simulink model "SWC_HALOUT_type"  (R2021b)
settings: Solver=FixedStepDiscrete  StartTime=0.0  StopTime=10.0  FixedStep=0.001  RelTol=1e-3
values from neighbouring files (symbols this model uses):
  DIDLen_APPPedalZP = uint16(3)    [vcu_local_hdr.m]
  DIDLen_APSFunConfig = uint16(16)    [vcu_local_hdr.m]
  DIDLen_AutoLock = uint16(1)    [vcu_local_hdr.m]
  DIDLen_AutoWipHSpdEN = uint16(1)    [vcu_local_hdr.m]
  DIDLen_DKCKey = uint16(8)    [vcu_local_hdr.m]
  DIDLen_DRLDis = uint16(1)    [vcu_local_hdr.m]
  DIDLen_DynoMode = uint16(1)    [vcu_local_hdr.m]
  DIDLen_FMHTimer = uint16(1)    [vcu_local_hdr.m]
  DIDLen_LFLowPresThre = uint16(1)    [vcu_local_hdr.m]
  DIDLen_LFSensorID = uint16(4)    [vcu_local_hdr.m]
  DIDLen_LRLowPresThre = uint16(1)    [vcu_local_hdr.m]
  DIDLen_LRSensorID = uint16(4)    [vcu_local_hdr.m]
  DIDLen_NVMPedalZP = uint16(3)    [vcu_local_hdr.m]
  DIDLen_RFLowPresThre = uint16(1)    [vcu_local_hdr.m]
  DIDLen_RFSensorID = uint16(4)    [vcu_local_hdr.m]
  DIDLen_RRLowPresThre = uint16(1)    [vcu_local_hdr.m]
  DIDLen_RRSensorID = uint16(4)    [vcu_local_hdr.m]
  DIDLen_SensorMode = uint16(1)    [vcu_local_hdr.m]
  DIDLen_TireSize = uint16(16)    [vcu_local_hdr.m]
  DIDLen_TPMSLearnSta = uint16(1)    [vcu_local_hdr.m]
  DIDLen_TurnLampFLThreCurr = uint16(1)    [vcu_local_hdr.m]
  DIDLen_TurnLampFRThreCurr = uint16(1)    [vcu_local_hdr.m]
  DIDLen_TurnLampRLThreCurr = uint16(1)    [vcu_local_hdr.m]
  DIDLen_TurnLampRRThreCurr = uint16(1)    [vcu_local_hdr.m]
  DIDLen_USSConfig = uint16(16)    [vcu_local_hdr.m]
  DIDLen_WhlPres = uint16(4)    [vcu_local_hdr.m]
  DIDLen_WhlSensorBattSta = uint16(1)    [vcu_local_hdr.m]
  DIDLen_WhlTmp = uint16(4)    [vcu_local_hdr.m]
  DIDLen_WipRLSCmdCutFilter = uint16(1)    [vcu_local_hdr.m]
  DIDLen_WipRLSCmdHoldFilter = uint16(1)    [vcu_local_hdr.m]
  DIDLen_XWDMode = uint16(1)    [vcu_local_hdr.m]
  DIDNum_APPPedalZP = uint16(0x0206)    [vcu_local_hdr.m]
  DIDNum_APSFunConfig = uint16(0x0903)    [vcu_local_hdr.m]
  DIDNum_AutoLock = uint16(0x0306)    [vcu_local_hdr.m]
  DIDNum_AutoWipHSpdEN = uint16(0x0308)    [vcu_local_hdr.m]
  DIDNum_DKCKey = uint16(0x0202)    [vcu_local_hdr.m]
  DIDNum_DRLDis = uint16(0x0307)    [vcu_local_hdr.m]
  DIDNum_DynoMode = uint16(0x0203)    [vcu_local_hdr.m]
  DIDNum_FMHTimer = uint16(0x0305)    [vcu_local_hdr.m]
  DIDNum_LFLowPresThre = uint16(0x0B08)    [vcu_local_hdr.m]
  DIDNum_LFSensorID = uint16(0x0B01)    [vcu_local_hdr.m]
  DIDNum_LRLowPresThre = uint16(0x0B0A)    [vcu_local_hdr.m]
  DIDNum_LRSensorID = uint16(0x0B03)    [vcu_local_hdr.m]
  DIDNum_NVMPedalZP = uint16(0x0207)    [vcu_local_hdr.m]
  DIDNum_RFLowPresThre = uint16(0x0B09)    [vcu_local_hdr.m]
  DIDNum_RFSensorID = uint16(0x0B02)    [vcu_local_hdr.m]
  DIDNum_RRLowPresThre = uint16(0x0B0B)    [vcu_local_hdr.m]
  DIDNum_RRSensorID = uint16(0x0B04)    [vcu_local_hdr.m]
  DIDNum_SensorMode = uint16(0x0B0C)    [vcu_local_hdr.m]
  DIDNum_TireSize = uint16(0x0902)    [vcu_local_hdr.m]
  DIDNum_TPMSLearnSta = uint16(0x0B0D)    [vcu_local_hdr.m]
  DIDNum_TurnLampFLThreCurr = uint16(0x0303)    [vcu_local_hdr.m]
  DIDNum_TurnLampFRThreCurr = uint16(0x0301)    [vcu_local_hdr.m]
  DIDNum_TurnLampRLThreCurr = uint16(0x0304)    [vcu_local_hdr.m]
  DIDNum_TurnLampRRThreCurr = uint16(0x0302)    [vcu_local_hdr.m]
  DIDNum_USSConfig = uint16(0x0901)    [vcu_local_hdr.m]
  DIDNum_WhlPres = uint16(0x0B05)    [vcu_local_hdr.m]
  DIDNum_WhlSensorBattSta = uint16(0x0B07)    [vcu_local_hdr.m]
  DIDNum_WhlTmp = uint16(0x0B06)    [vcu_local_hdr.m]
  DIDNum_WipRLSCmdCutFilter = uint16(0x030A)    [vcu_local_hdr.m]
  DIDNum_WipRLSCmdHoldFilter = uint16(0x0309)    [vcu_local_hdr.m]
  DIDNum_XWDMode = uint16(0x0201)    [vcu_local_hdr.m]
  ENUM_TPMSLearnStatus_LEARNED = uint8(  1  )    [vcu_local_hdr.m]
  ENUM_TPMSLearnStatus_LEARNFAIL = uint8(  2  )    [vcu_local_hdr.m]
  ENUM_TPMSLearnStatus_NOTLEARN = uint8(  0  )    [vcu_local_hdr.m]
  FALSE = boolean( 0 )    [vcu_local_hdr.m]    (also in vcu_local_hdrTA2.m)
  TRUE = boolean( 1 )    [vcu_local_hdr.m]    (also in vcu_local_hdrTA2.m)
  ZERO_INT = uint8(0)    [vcu_local_hdr.m]    (also in vcu_local_hdrTA2.m)
undefined symbols (not defined in the file or in its folder): f32_ApsOutVehSpdSig, R_DIDWriteCDD_CSOP_DIDSet_APPPedalZP, R_DIDWriteCDD_CSOP_DIDSet_APSFunConfig, R_DIDWriteCDD_CSOP_DIDSet_AutoLock, R_DIDWriteCDD_CSOP_DIDSet_AutoWipHSpdEN, R_DIDWriteCDD_CSOP_DIDSet_DKCKey, R_DIDWriteCDD_CSOP_DIDSet_DRLDis, R_DIDWriteCDD_CSOP_DIDSet_DynoMode, R_DIDWriteCDD_CSOP_DIDSet_FMHTimer, R_DIDWriteCDD_CSOP_DIDSet_LFLowPresThre, R_DIDWriteCDD_CSOP_DIDSet_LFSensorID, R_DIDWriteCDD_CSOP_DIDSet_LRLowPresThre, R_DIDWriteCDD_CSOP_DIDSet_LRSensorID, R_DIDWriteCDD_CSOP_DIDSet_NVMPedalZP, R_DIDWriteCDD_CSOP_DIDSet_RFLowPresThre, R_DIDWriteCDD_CSOP_DIDSet_RFSensorID, R_DIDWriteCDD_CSOP_DIDSet_RRLowPresThre, R_DIDWriteCDD_CSOP_DIDSet_RRSensorID, R_DIDWriteCDD_CSOP_DIDSet_SensorMode, R_DIDWriteCDD_CSOP_DIDSet_TireSize, R_DIDWriteCDD_CSOP_DIDSet_TPMSLearnSta, R_DIDWriteCDD_CSOP_DIDSet_TurnLampFLThreCurr, R_DIDWriteCDD_CSOP_DIDSet_TurnLampFRThreCurr, R_DIDWriteCDD_CSOP_DIDSet_TurnLampRLThreCurr, R_DIDWriteCDD_CSOP_DIDSet_TurnLampRRThreCurr, R_DIDWriteCDD_CSOP_DIDSet_USSConfig, R_DIDWriteCDD_CSOP_DIDSet_WhlPres, R_DIDWriteCDD_CSOP_DIDSet_WhlSensorBattSta, R_DIDWriteCDD_CSOP_DIDSet_WhlTmp, R_DIDWriteCDD_CSOP_DIDSet_WipRLSCmdCutFilter, R_DIDWriteCDD_CSOP_DIDSet_WipRLSCmdHoldFilter, R_DIDWriteCDD_CSOP_DIDSet_XWDMode, R_FDCCDD_Inner_CSOP_FDC_AppCallSleep, R_HALINCDD_CSOP_PAS_Handler, R_HALINCDD_CSOP_UDS_Main, R_HALOUT_APS_CSOP_ApsOutput, R_HALOUTCDD_CSOP_AppNmStateReq, R_HALOUTCDD_CSOP_ResetPedalZeroPosDone, R_HALOUTCDD_CSOP_SetAcoreRebootCmdACK, R_HALOUTCDD_CSOP_SetHazardIND, R_HALOUTCDD_CSOP_SetSysPwrStat, R_HALOUTCDD_CSOP_SleepRequest, R_HALOUTCDD_CSOP_TPMSSensorIDRegSetResults, R_IOExpOUT_CDD_CSOP_IOExpSetVal, R_J1939_CAN1_FD1_CE100_0_CSOP_Write_CAN1_FD1_CE100_0, R_J1939_CAN1_FD1_CE100_1_CSOP_Write_CAN1_FD1_CE100_1, R_NVMWriteCDD_Inner_NVM_WriteOperation, R_UDSCDD_CSOP_DdmRestartOperationCycle, R_WDGCDD_CSOP_Call_WDG_AppEnd, u16_DIDLen_APPPedalZP, u16_DIDLen_APSFunConfig, u16_DIDLen_AutoLock, u16_DIDLen_AutoWipHSpdEN, u16_DIDLen_DKCKey, u16_DIDLen_DRLDis, u16_DIDLen_DynoMode, u16_DIDLen_FMHTimer, u16_DIDLen_LFLowPresThre, u16_DIDLen_LFSensorID, u16_DIDLen_LRLowPresThre ... (+95)
libraries: FVT_lib x142, simulink x107, hdlsllib x6, hcu_lib x5, halout x1
(part 6 of 8)

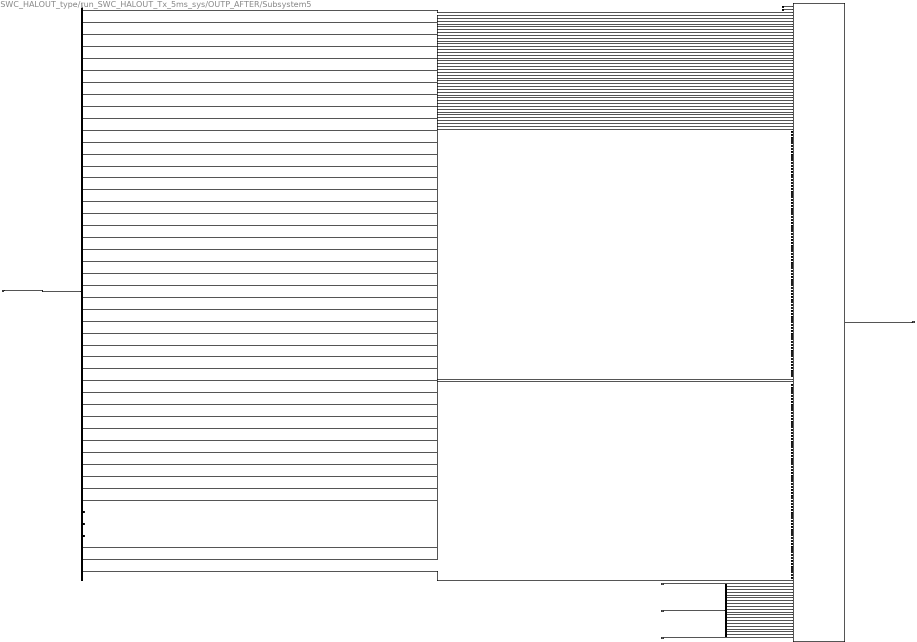
== system SWC_HALOUT_type/run_SWC_HALOUT_Tx_5ms_sys/OUTP_AFTER/Subsystem5 ==
  BOUTP_outputs : Inport
  BHAL_SYSTPMS_outputs : Inport  Port=2
  BHAL_SYS_outputs : Inport  Port=3
  BHAL_DIDGetData_raw : Inport  Port=4
  Bus Selector : BusSelector  OutputSignals=VOUTP_WriteChkLFID_raw,VOUTP_WriteChkRFID_raw,VOUTP_WriteChkLRID_raw,VOUTP_WriteChkRRID_raw,VOUTP_WriteChkfinLFID_raw,VOUTP_WriteChkfinRFID_raw,VOUTP_WriteChkfinLRID_raw,VOUTP_WriteChkfinRRID_raw,VOUTP_LFSensorFail_flg,VOUTP_RFSensorFail_flg,VOUTP_LRSensorFail_flg,VOUTP_RRSensorFail_flg,VOUTP_LFWheelPSW_raw8,VOUTP_RFWheelPSW_raw8,VOUTP_LRWheelPSW_raw8,VOUTP_RRWheelPSW_raw8,VOUTP_LFPindi_enum,VOUTP_RFPind_enum,VOUTP_LRPindi_enum,VOUTP_RRPindi_enum,VOUTP_LFP20_raw8,VOUTP_RFP20_raw8,VOUTP_LRP20_raw8,VOUTP_RRP20_raw8,VOUTP_LFWheelPress_raw8,VOUTP_RFWheelPress_raw8,VOUTP_LRWheelPress_raw8,VOUTP_RRWheelPress_raw8,VOUTP_LFWheelTemp_C,VOUTP_RFWheelTemp_C,VOUTP_LRWheelTemp_C,VOUTP_RRWheelTemp_C,VOUTP_Flashchkdatavalid_enum,VOUTP_Flashdatavalid_enum,VOUTP_unlearnSfali_flg,VOUTP_unlearnSfailvalid_enum,VOUTP_Prepresstempvalid_enum,VOUTP_FlashS1ID_raw,VOUTP_FlashS2ID_raw,VOUTP_FlashS3ID_raw,VOUTP_FlashS4ID_raw,VOUTP_FlashIDvalid_enum,VOUTP_EAPS1MIN_pct,VOUTP_EAPS2MIN_pct,VOUTP_SaveRegenMode_enum,VOUTP_ModelVersion_raw,VOUTP_ModelVersionChksum_raw,VOUTP_JudgeKeepUnlockZone_flg
  Bus Selector1 : BusSelector  OutputSignals=VHAL_RandomnumberY_raw1,VHAL_RandomnumberY_raw2,VHAL_RandomnumberY_raw3,VHAL_RandomnumberY_raw4,VHAL_RandomnumberY_raw5,VHAL_RandomnumberY_raw6,VHAL_RandomnumberY_raw7,VHAL_RandomnumberY_raw8,VHAL_funAuto_flg,VHAL_DiagDRLOFF_flg,VHAL_DiagFMHT_s,VHAL_DiagFLTC_mA,VHAL_DiagFRTC_mA,VHAL_DiagRLTC_mA,VHAL_DiagRRTC_mA,VHAL_USSConfig_raw8,VHAL_TireSize_raw8,VHAL_APSFunConfig_raw8
  Enabled Subsystem : Subsystem  TreatAsAtomicUnit=on
  Ground : Ground
  Ground1 : Ground
  Ground_{3..158} (156 alike) : Ground
  Terminator_1 : Terminator
  Terminator_2 : Terminator
  Terminator_3 : Terminator
  HAL_NvmWriteData_raw : Outport
  wires:
  BOUTP_outputs/1 -> Bus Selector/1
  Enabled Subsystem/1(HAL_NvmWriteData_raw) -> HAL_NvmWriteData_raw/1
  Bus Selector1/2 -> Enabled Subsystem/206(VHAL_RandomnumberY_raw2)  "<VHAL_RandomnumberY_raw2>"
  Bus Selector1/3 -> Enabled Subsystem/207(VHAL_RandomnumberY_raw3)  "<VHAL_RandomnumberY_raw3>"
  Bus Selector1/4 -> Enabled Subsystem/208(VHAL_RandomnumberY_raw4)  "<VHAL_RandomnumberY_raw4>"
  Bus Selector1/5 -> Enabled Subsystem/209(VHAL_RandomnumberY_raw5)  "<VHAL_RandomnumberY_raw5>"
  Bus Selector1/6 -> Enabled Subsystem/210(VHAL_RandomnumberY_raw6)  "<VHAL_RandomnumberY_raw6>"
  Bus Selector1/7 -> Enabled Subsystem/211(VHAL_RandomnumberY_raw7)  "<VHAL_RandomnumberY_raw7>"
  Bus Selector1/8 -> Enabled Subsystem/212(VHAL_RandomnumberY_raw8)  "<VHAL_RandomnumberY_raw8>"
  Bus Selector/22 -> Enabled Subsystem/24(VOUTP_RFP20_raw8)  "<VOUTP_RFP20_raw8>"
  Bus Selector/21 -> Enabled Subsystem/23(VOUTP_LFP20_raw8)  "<VOUTP_LFP20_raw8>"
  Bus Selector/23 -> Enabled Subsystem/25(VOUTP_LRP20_raw8)  "<VOUTP_LRP20_raw8>"
  Bus Selector/20 -> Enabled Subsystem/22(VOUTP_RRPindi_enum)  "<VOUTP_RRPindi_enum>"
  Bus Selector/24 -> Enabled Subsystem/26(VOUTP_RRP20_raw8)  "<VOUTP_RRP20_raw8>"
  Bus Selector/19 -> Enabled Subsystem/21(VOUTP_LRPindi_enum)  "<VOUTP_LRPindi_enum>"
  Bus Selector/25 -> Enabled Subsystem/27(VOUTP_LFWheelPress_raw8)  "<VOUTP_LFWheelPress_raw8>"
  Bus Selector/18 -> Enabled Subsystem/20(VOUTP_RFPindi_enum)  "<VOUTP_RFPind_enum>"
  Bus Selector/26 -> Enabled Subsystem/28(VOUTP_RFWheelPress_raw8)  "<VOUTP_RFWheelPress_raw8>"
  Bus Selector/17 -> Enabled Subsystem/19(VOUTP_LFPindi_enum)  "<VOUTP_LFPindi_enum>"
  Bus Selector/27 -> Enabled Subsystem/29(VOUTP_LRWheelPress_raw8)  "<VOUTP_LRWheelPress_raw8>"
  Bus Selector/16 -> Enabled Subsystem/18(VOUTP_RRWheelPSW_raw8)  "<VOUTP_RRWheelPSW_raw8>"
  Bus Selector/28 -> Enabled Subsystem/30(VOUTP_RRWheelPress_raw8)  "<VOUTP_RRWheelPress_raw8>"
  Bus Selector/15 -> Enabled Subsystem/17(VOUTP_LRWheelPSW_raw8)  "<VOUTP_LRWheelPSW_raw8>"
  Bus Selector/29 -> Enabled Subsystem/31(VOUTP_LFWheelTemp_C)  "<VOUTP_LFWheelTemp_C>"
  Bus Selector/14 -> Enabled Subsystem/16(VOUTP_RFWheelPSW_raw8)  "<VOUTP_RFWheelPSW_raw8>"
  Bus Selector/30 -> Enabled Subsystem/32(VOUTP_RFWheelTemp_C)  "<VOUTP_RFWheelTemp_C>"
  Bus Selector/13 -> Enabled Subsystem/15(VOUTP_LFWheelPSW_raw8)  "<VOUTP_LFWheelPSW_raw8>"
  Bus Selector/31 -> Enabled Subsystem/33(VOUTP_LRWheelTemp_C)  "<VOUTP_LRWheelTemp_C>"
  Bus Selector/12 -> Enabled Subsystem/14(VOUTP_RRSensorFail_flg)  "<VOUTP_RRSensorFail_flg>"
  Bus Selector/32 -> Enabled Subsystem/34(VOUTP_RRWheelTemp_C)  "<VOUTP_RRWheelTemp_C>"
  Bus Selector/11 -> Enabled Subsystem/13(VOUTP_LRSensorFail_flg)  "<VOUTP_LRSensorFail_flg>"
  Bus Selector/33 -> Enabled Subsystem/35(VOUTP_Flashchkdatavalid_enum)  "<VOUTP_Flashchkdatavalid_enum>"
  Bus Selector/10 -> Enabled Subsystem/12(VOUTP_RFSensorFail_flg)  "<VOUTP_RFSensorFail_flg>"
  Bus Selector/34 -> Enabled Subsystem/36(VOUTP_Flashdatavalid_enum)  "<VOUTP_Flashdatavalid_enum>"
  Bus Selector/9 -> Enabled Subsystem/11(VOUTP_LFSensorFail_flg)  "<VOUTP_LFSensorFail_flg>"
  Bus Selector/35 -> Enabled Subsystem/37(VOUTP_unlearnSfali_flg)  "<VOUTP_unlearnSfali_flg>"
  Bus Selector/36 -> Enabled Subsystem/38(VOUTP_unlearnSfailvalid_enum)  "<VOUTP_unlearnSfailvalid_enum>"
  Bus Selector/37 -> Enabled Subsystem/39(VOUTP_Prepresstempvalid_enum)  "<VOUTP_Prepresstempvalid_enum>"
  BHAL_SYSTPMS_outputs/1 -> Enabled Subsystem/204(BHAL_SYSTPMS_outputs)
  Bus Selector/8 -> Enabled Subsystem/10(VOUTP_WriteChkfinRRID_raw)  "<VOUTP_WriteChkfinRRID_raw>"
  Bus Selector/7 -> Enabled Subsystem/9(VOUTP_WriteChkfinLRID_raw)  "<VOUTP_WriteChkfinLRID_raw>"
  Bus Selector/6 -> Enabled Subsystem/8(VOUTP_WriteChkfinRFID_raw)  "<VOUTP_WriteChkfinRFID_raw>"
  Bus Selector/5 -> Enabled Subsystem/7(VOUTP_WriteChkfinLFID_raw)  "<VOUTP_WriteChkfinLFID_raw>"
  Bus Selector/4 -> Enabled Subsystem/6(VOUTP_WriteChkRRID_raw)  "<VOUTP_WriteChkRRID_raw>"
  Bus Selector/3 -> Enabled Subsystem/5(VOUTP_WriteChkLRID_raw)  "<VOUTP_WriteChkLRID_raw>"
  Bus Selector/2 -> Enabled Subsystem/4(VOUTP_WriteChkRFID_raw)  "<VOUTP_WriteChkRFID_raw>"
  Bus Selector/1 -> Enabled Subsystem/3(VOUTP_WriteChkLFID_raw)  "<VOUTP_WriteChkLFID_raw>"
  Bus Selector1/1 -> Enabled Subsystem/205(VHAL_RandomnumberY_raw1)  "<VHAL_RandomnumberY_raw1>"
  Bus Selector/38 -> Enabled Subsystem/40(VOUTP_FlashS1ID_raw)  "<VOUTP_FlashS1ID_raw>"
  Bus Selector/39 -> Enabled Subsystem/41(VOUTP_FlashS2ID_raw)  "<VOUTP_FlashS2ID_raw>"
  Bus Selector/40 -> Enabled Subsystem/42(VOUTP_FlashS3ID_raw)  "<VOUTP_FlashS3ID_raw>"
  Bus Selector/41 -> Enabled Subsystem/43(VOUTP_FlashS41ID_raw)  "<VOUTP_FlashS4ID_raw>"
  Bus Selector/42 -> Enabled Subsystem/44(VOUTP_FlashIDvalid_enum)  "<VOUTP_FlashIDvalid_enum>"
  BHAL_SYS_outputs/1 -> Bus Selector1/1
  Bus Selector1/9 -> Enabled Subsystem/213(VHAL_funAuto_flg)  "<VHAL_funAuto_flg>"
  Bus Selector1/10 -> Enabled Subsystem/214(VHAL_DiagDRLOFF_flg)  "<VHAL_DiagDRLOFF_flg>"
  Bus Selector1/11 -> Enabled Subsystem/215(VHAL_DiagFMHT_s)  "<VHAL_DiagFMHT_s>"
  Bus Selector1/12 -> Enabled Subsystem/216(VHAL_DiagFLTC_mA)  "<VHAL_DiagFLTC_mA>"
  Bus Selector1/13 -> Enabled Subsystem/217(VHAL_DiagFRTC_mA)  "<VHAL_DiagFRTC_mA>"
  Bus Selector1/14 -> Enabled Subsystem/218(VHAL_DiagRLTC_mA)  "<VHAL_DiagRLTC_mA>"
  Bus Selector1/15 -> Enabled Subsystem/219(VHAL_DiagRRTC_mA)  "<VHAL_DiagRRTC_mA>"
  Bus Selector1/16 -> Enabled Subsystem/220(VHAL_USSConfig_raw8)  "<VHAL_USSConfig_raw8>"
  Bus Selector1/17 -> Enabled Subsystem/221(VHAL_TireSize_raw8)  "<VHAL_TireSize_raw8>"
  Bus Selector1/18 -> Enabled Subsystem/222(VHAL_APSFunConfig_raw8)  "<VHAL_APSFunConfig_raw8>"
  BHAL_DIDGetData_raw/1 -> Enabled Subsystem/223(BHAL_DIDGetData_raw)
  Bus Selector/46 -> Enabled Subsystem/132(VOUTP_ModelVersion_raw)  "<VOUTP_ModelVersion_raw>"
  Bus Selector/47 -> Enabled Subsystem/133(VOUTP_ModelVersionChksum_raw)  "<VOUTP_ModelVersionChksum_raw>"
  Bus Selector/48 -> Enabled Subsystem/203(VOUTP_JudgeKeepUnlockZone_flg)  "<VOUTP_JudgeKeepUnlockZone_flg>"
  Ground/1 -> Enabled Subsystem/2(VOUTP_DrivetrainSelect_enum)
  Ground1/1 -> Enabled Subsystem/1(VOUTP_AntitheftSta_enum)
  Bus Selector/43 -> Terminator_1/1  "<VOUTP_EAPS1MIN_pct>"
  Bus Selector/44 -> Terminator_2/1  "<VOUTP_EAPS2MIN_pct>"
  Bus Selector/45 -> Terminator_3/1  "<VOUTP_SaveRegenMode_enum>"
  Ground_3/1 -> Enabled Subsystem/45(VOUTP_ACModeMem_enum)
  Ground_4/1 -> Enabled Subsystem/46(VOUTP_Face_flg)
  Ground_5/1 -> Enabled Subsystem/47(VOUTP_Foot_flg)
  Ground_6/1 -> Enabled Subsystem/48(VOUTP_Frost_flg)
  Ground_7/1 -> Enabled Subsystem/49(VOUTP_FaceM_flg)
  Ground_8/1 -> Enabled Subsystem/50(VOUTP_FootM_flg)
  Ground_9/1 -> Enabled Subsystem/51(VOUTP_CCUSyncSts_flg)
  Ground_10/1 -> Enabled Subsystem/52(VOUTP_ACForceOFF_flg)
  Ground_11/1 -> Enabled Subsystem/53(VOUTP_sigRecircSt_flg)
  Ground_12/1 -> Enabled Subsystem/54(VOUTP_RecAutoFlg_flg)
  Ground_13/1 -> Enabled Subsystem/55(VOUTP_AirIntenZone1M_enum)
  Ground_14/1 -> Enabled Subsystem/56(VOUTP_fdefog_flg)
  Ground_15/1 -> Enabled Subsystem/57(VOUTP_sigSetTempZon1St_C)
  Ground_16/1 -> Enabled Subsystem/58(VOUTP_sigSetTempZon2StM_C)
  Ground_17/1 -> Enabled Subsystem/59(VOUT_CountAlarm_enum)
  Ground_18/1 -> Enabled Subsystem/60(VOUTP_MFSWTri_flg)
  Ground_19/1 -> Enabled Subsystem/61(VOUTP_MirrorFlodPos_flg)
  Ground_20/1 -> Enabled Subsystem/62(VOUTP_FuelDoorPos_flg)
  Ground_21/1 -> Enabled Subsystem/63(VOUTP_LockSetting_flg)
  Ground_22/1 -> Enabled Subsystem/64(VOUTP_MFRDNBrightReq_pct)
  Ground_23/1 -> Enabled Subsystem/65(VOUTP_RoomLampMode_flg)
  Ground_24/1 -> Enabled Subsystem/66(VOUTP_WiperFixMode_flg)
  Ground_25/1 -> Enabled Subsystem/67(VOUTP_IVIPTGUSStaSW_flg)
  Ground_26/1 -> Enabled Subsystem/68(VOUTP_EAPS1MIN_pct)
  Ground_27/1 -> Enabled Subsystem/69(VOUTP_EAPS2MIN_pct)
  Ground_28/1 -> Enabled Subsystem/70(VOUTP_HoodSW_flg)
  Ground_29/1 -> Enabled Subsystem/71(VOUTP_TailgateSW_flg)
  Ground_30/1 -> Enabled Subsystem/72(VOUTP_CTDLockSW_flg)
  Ground_31/1 -> Enabled Subsystem/73(VOUTP_TailgateHDSW_flg)
  Ground_32/1 -> Enabled Subsystem/74(VOUTP_APMDoorControlSta_flg)
  Ground_33/1 -> Enabled Subsystem/75(VOUTP_fUnlockSingle_flg)
  Ground_34/1 -> Enabled Subsystem/76(VOUTP_SaveRegenMode_enum)
  Ground_35/1 -> Enabled Subsystem/77(VOUTP_AmbFunENFlash_enum)
  Ground_36/1 -> Enabled Subsystem/78(VOUTP_AmbWelENFlash_enum)
  Ground_37/1 -> Enabled Subsystem/79(VOUTP_AmbDimENFlash_enum)
  Ground_38/1 -> Enabled Subsystem/80(VOUTP_AmbLinkDriStaFlash_enum)
  Ground_39/1 -> Enabled Subsystem/81(VOUTP_AmbPwrWarnENFlash_enum)
  Ground_40/1 -> Enabled Subsystem/82(VOUTP_AmbODAENFlash_enum)
  Ground_41/1 -> Enabled Subsystem/83(VOUTP_AmbColorSta1_enum)
  Ground_42/1 -> Enabled Subsystem/84(VOUTP_AmbColorSta2_enum)
  Ground_43/1 -> Enabled Subsystem/85(VOUTP_AmbColorSta3_enum)
  Ground_44/1 -> Enabled Subsystem/86(VOUTP_AmbColorSta4_enum)
  Ground_45/1 -> Enabled Subsystem/87(VOUTP_AmbColorSta5_enum)
  Ground_46/1 -> Enabled Subsystem/88(VOUTP_AmbColorSta7_enum)
  Ground_47/1 -> Enabled Subsystem/89(VOUTP_AmbBrightnessSta1_enum)
  Ground_48/1 -> Enabled Subsystem/90(VOUTP_AmbBrightnessSta2_enum)
  Ground_49/1 -> Enabled Subsystem/91(VOUTP_AmbBrightnessSta3_enum)
  Ground_50/1 -> Enabled Subsystem/92(VOUTP_AmbBrightnessSta4_enum)
  Ground_51/1 -> Enabled Subsystem/93(VOUTP_AmbBrightnessSta5_enum)
  Ground_52/1 -> Enabled Subsystem/94(VOUTP_AmbBrightnessSta7_enum)
  Ground_53/1 -> Enabled Subsystem/95(VOUTP_TurnSwTimeSetSta123_enum)
  Ground_54/1 -> Enabled Subsystem/96(VOUTP_TurnSwTimeSetSta457_enum)
  Ground_55/1 -> Enabled Subsystem/97(VOUTP_FDCTHCAirIntZ3Sta_enum)
  Ground_56/1 -> Enabled Subsystem/98(VOUTP_FDCTHCPsEVentModeSta_enum)
  Ground_57/1 -> Enabled Subsystem/99(VOUTP_FDCTHCDrEVentModeSta_enum)
  Ground_58/1 -> Enabled Subsystem/100(VOUTP_FDCTHCDrEVentZSta_enum)
  Ground_59/1 -> Enabled Subsystem/101(VOUTP_FDCTHCCLEVentZSta_enum)
  Ground_60/1 -> Enabled Subsystem/102(VOUTP_FDCTHCPsEVentZSta_enum)
  Ground_61/1 -> Enabled Subsystem/103(VOUTP_FDCTHCCREVentZSta_enum)
  Ground_62/1 -> Enabled Subsystem/104(VOUTP_DrVentEN_flg)
  Ground_63/1 -> Enabled Subsystem/105(VOUTP_FDCTHCDrEVentYSta_enum)
  Ground_64/1 -> Enabled Subsystem/106(VOUTP_CLVentEN_flg)
  Ground_65/1 -> Enabled Subsystem/107(VOUTP_FDCTHCCLEVentYSta_enum)
  Ground_66/1 -> Enabled Subsystem/108(VOUTP_PsVentEN_flg)
  Ground_67/1 -> Enabled Subsystem/109(VOUTP_FDCTHCPsEVentYSta_enum)
  Ground_68/1 -> Enabled Subsystem/110(VOUTP_CRVentEN_flg)
  Ground_69/1 -> Enabled Subsystem/111(VOUTP_FDCTHCCREVentYSta_enum)
  Ground_70/1 -> Enabled Subsystem/112(VOUTP_FDCFGSAirIntSta_enum)
  Ground_71/1 -> Enabled Subsystem/113(VOUTP_FDCFGSChSta_enum)
  Ground_72/1 -> Enabled Subsystem/114(VOUTP_FDCFGSIONSWSta_flg)
  Ground_73/1 -> Enabled Subsystem/115(VOUTP_WalkOutLkENFunSta_flg)
  Ground_74/1 -> Enabled Subsystem/116(VOUTP_WalkInUnLkENFunSta_flg)
  Ground_75/1 -> Enabled Subsystem/117(VOUTP_FollowMeENFunSta_flg)
  Ground_76/1 -> Enabled Subsystem/118(VOUTP_PTGUserHeight1_cnt)
  Ground_77/1 -> Enabled Subsystem/119(VOUTP_PTGUserHeight2_cnt)
  Ground_78/1 -> Enabled Subsystem/120(VOUTP_PTGUserHeight3_cnt)
  Ground_79/1 -> Enabled Subsystem/121(VOUTP_PTGUserHeight4_cnt)
  Ground_80/1 -> Enabled Subsystem/122(VOUTP_PTGUserHeight5_cnt)
  Ground_81/1 -> Enabled Subsystem/123(VOUTP_PTGUserHeight7_cnt)
  Ground_82/1 -> Enabled Subsystem/124(VOUTP_PTGOpenHeight12_enum)
  Ground_83/1 -> Enabled Subsystem/125(VOUTP_PTGOpenHeight34_enum)
  Ground_84/1 -> Enabled Subsystem/126(VOUTP_PTGOpenHeight57_enum)
  Ground_85/1 -> Enabled Subsystem/127(VOUTP_ACCLevelMem12_enum)
  Ground_86/1 -> Enabled Subsystem/128(VOUTP_ACCLevelMem34_enum)
  Ground_87/1 -> Enabled Subsystem/129(VOUTP_ACCLevelMem57_enum)
  Ground_88/1 -> Enabled Subsystem/130(VOUTP_AutoLockMem_enum)
  Ground_89/1 -> Enabled Subsystem/131(VOUTP_AutoUnlockMem_enum)
  Ground_90/1 -> Enabled Subsystem/134(VOUTP_HMIKey1FuncSta_enum)
  Ground_91/1 -> Enabled Subsystem/135(VOUTP_HMIKey2FuncSta_enum)
  Ground_92/1 -> Enabled Subsystem/136(VOUTP_HMIKey3FuncSta_enum)
  Ground_93/1 -> Enabled Subsystem/137(VOUTP_HMIKey4FuncSta_enum)
  Ground_94/1 -> Enabled Subsystem/138(VOUTP_HMIKey5FuncSta_enum)
  Ground_95/1 -> Enabled Subsystem/139(VOUTP_HMIKey6FuncSta_enum)
  Ground_96/1 -> Enabled Subsystem/140(VOUTP_HMIKey7FuncSta_enum)
  Ground_97/1 -> Enabled Subsystem/141(VOUTP_HMIKey8FuncSta_enum)
  Ground_98/1 -> Enabled Subsystem/142(VOUTP_AutoWipHSpdENSta_flg)
  Ground_99/1 -> Enabled Subsystem/143(VOUTP_AirIntenZone1MSet2_enum)
  Ground_100/1 -> Enabled Subsystem/144(VOUTP_AirIntenZone1MSet3_enum)
  Ground_101/1 -> Enabled Subsystem/145(VOUTP_AirIntenZone1MSet4_enum)
  Ground_102/1 -> Enabled Subsystem/146(VOUTP_AirIntenZone1MSet5_enum)
  Ground_103/1 -> Enabled Subsystem/147(VOUTP_AirIntenZone1MSet7_enum)
  Ground_104/1 -> Enabled Subsystem/148(VOUTP_AirIntenZone3MSet2_enum)
  Ground_105/1 -> Enabled Subsystem/149(VOUTP_AirIntenZone3MSet3_enum)
  Ground_106/1 -> Enabled Subsystem/150(VOUTP_AirIntenZone3MSet4_enum)
  Ground_107/1 -> Enabled Subsystem/151(VOUTP_AirIntenZone3MSet5_enum)
  Ground_108/1 -> Enabled Subsystem/152(VOUTP_AirIntenZone3MSet7_enum)
  Ground_109/1 -> Enabled Subsystem/153(VOUTP_FDCFGSChStaSet457_enum)
  Ground_110/1 -> Enabled Subsystem/154(VOUTP_FDCFGSAirIntStaSet457_enum)
  Ground_111/1 -> Enabled Subsystem/155(VOUTP_DrEVentModeStaSet457_enum)
  Ground_112/1 -> Enabled Subsystem/156(VOUTP_PsEVentModeStaSet457_enum)
  Ground_113/1 -> Enabled Subsystem/157(VOUTP_FDCTHCDrEVentZStaSet2_enum)
  Ground_114/1 -> Enabled Subsystem/158(VOUTP_FDCTHCDrEVentZStaSet3_enum)
  Ground_115/1 -> Enabled Subsystem/159(VOUTP_FDCTHCDrEVentZStaSet4_enum)
  Ground_116/1 -> Enabled Subsystem/160(VOUTP_FDCTHCDrEVentZStaSet5_enum)
  Ground_117/1 -> Enabled Subsystem/161(VOUTP_FDCTHCDrEVentZStaSet7_enum)
  Ground_118/1 -> Enabled Subsystem/162(VOUTP_FDCTHCCLEVentZStaSet2_enum)
  Ground_119/1 -> Enabled Subsystem/163(VOUTP_FDCTHCCLEVentZStaSet3_enum)
  Ground_120/1 -> Enabled Subsystem/164(VOUTP_FDCTHCCLEVentZStaSet4_enum)
  Ground_121/1 -> Enabled Subsystem/165(VOUTP_FDCTHCCLEVentZStaSet5_enum)
  Ground_122/1 -> Enabled Subsystem/166(VOUTP_FDCTHCCLEVentZStaSet7_enum)
  Ground_123/1 -> Enabled Subsystem/167(VOUTP_FDCTHCPsEVentZStaSet2_enum)
  Ground_124/1 -> Enabled Subsystem/168(VOUTP_FDCTHCPsEVentZStaSet3_enum)
  Ground_125/1 -> Enabled Subsystem/169(VOUTP_FDCTHCPsEVentZStaSet4_enum)
  Ground_126/1 -> Enabled Subsystem/170(VOUTP_FDCTHCPsEVentZStaSet5_enum)
  Ground_127/1 -> Enabled Subsystem/171(VOUTP_FDCTHCPsEVentZStaSet7_enum)
  Ground_128/1 -> Enabled Subsystem/172(VOUTP_FDCTHCCREVentZStaSet2_enum)
  Ground_129/1 -> Enabled Subsystem/173(VOUTP_FDCTHCCREVentZStaSet3_enum)
  Ground_130/1 -> Enabled Subsystem/174(VOUTP_FDCTHCCREVentZStaSet4_enum)
  Ground_131/1 -> Enabled Subsystem/175(VOUTP_FDCTHCCREVentZStaSet5_enum)
  Ground_132/1 -> Enabled Subsystem/176(VOUTP_FDCTHCCREVentZStaSet7_enum)
  Ground_133/1 -> Enabled Subsystem/177(VOUTP_FDCTHCDrEVentYStaSet2_enum)
  Ground_134/1 -> Enabled Subsystem/178(VOUTP_FDCTHCDrEVentYStaSet3_enum)
  Ground_135/1 -> Enabled Subsystem/179(VOUTP_FDCTHCDrEVentYStaSet4_enum)
  Ground_136/1 -> Enabled Subsystem/180(VOUTP_FDCTHCDrEVentYStaSet5_enum)
  Ground_137/1 -> Enabled Subsystem/181(VOUTP_FDCTHCDrEVentYStaSet7_enum)
  Ground_138/1 -> Enabled Subsystem/182(VOUTP_FDCTHCCLEVentYStaSet2_enum)
  Ground_139/1 -> Enabled Subsystem/183(VOUTP_FDCTHCCLEVentYStaSet3_enum)
  Ground_140/1 -> Enabled Subsystem/184(VOUTP_FDCTHCCLEVentYStaSet4_enum)
  Ground_141/1 -> Enabled Subsystem/185(VOUTP_FDCTHCCLEVentYStaSet5_enum)
  Ground_142/1 -> Enabled Subsystem/186(VOUTP_FDCTHCCLEVentYStaSet7_enum)
  Ground_143/1 -> Enabled Subsystem/187(VOUTP_FDCTHCPsEVentYStaSet2_enum)
  Ground_144/1 -> Enabled Subsystem/188(VOUTP_FDCTHCPsEVentYStaSet3_enum)
  Ground_145/1 -> Enabled Subsystem/189(VOUTP_FDCTHCPsEVentYStaSet4_enum)
  Ground_146/1 -> Enabled Subsystem/190(VOUTP_FDCTHCPsEVentYStaSet5_enum)
  Ground_147/1 -> Enabled Subsystem/191(VOUTP_FDCTHCPsEVentYStaSet7_enum)
  Ground_148/1 -> Enabled Subsystem/192(VOUTP_FDCTHCCREVentYStaSet2_enum)
  Ground_149/1 -> Enabled Subsystem/193(VOUTP_FDCTHCCREVentYStaSet3_enum)
  Ground_150/1 -> Enabled Subsystem/194(VOUTP_FDCTHCCREVentYStaSet4_enum)
  Ground_151/1 -> Enabled Subsystem/195(VOUTP_FDCTHCCREVentYStaSet5_enum)
  Ground_152/1 -> Enabled Subsystem/196(VOUTP_FDCTHCCREVentYStaSet7_enum)
  Ground_153/1 -> Enabled Subsystem/197(VOUTP_ACModeSet457_enum)
  Ground_154/1 -> Enabled Subsystem/198(VOUTP_SettempZon1Set2_enum)
  Ground_155/1 -> Enabled Subsystem/199(VOUTP_SettempZon1Set3_enum)
  Ground_156/1 -> Enabled Subsystem/200(VOUTP_SettempZon1Set4_enum)
  Ground_157/1 -> Enabled Subsystem/201(VOUTP_SettempZon1Set5_enum)
  Ground_158/1 -> Enabled Subsystem/202(VOUTP_SettempZon1Set7_enum)

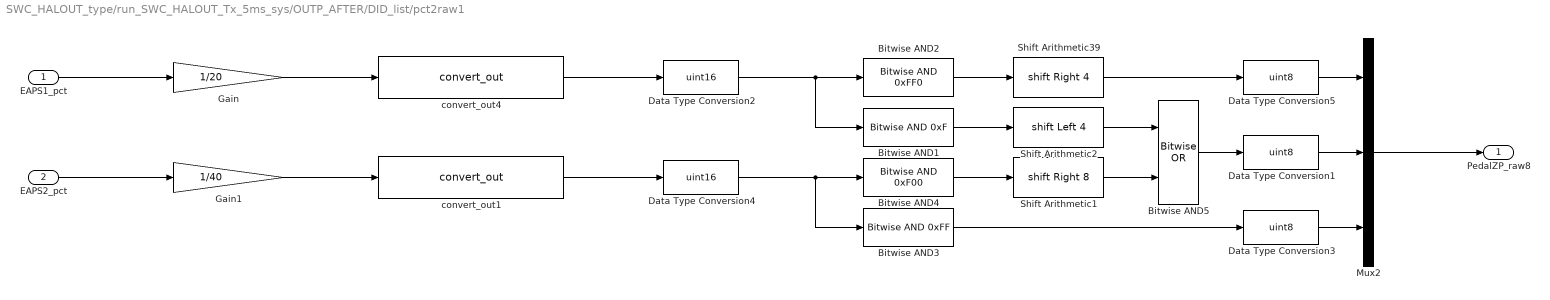
== system SWC_HALOUT_type/run_SWC_HALOUT_Tx_5ms_sys/OUTP_AFTER/DID_list/pct2raw1 ==
  EAPS1_pct : Inport
  EAPS2_pct : Inport  Port=2
  Bitwise AND1 : simulink/Logic and Bit Operations/Bitwise Operator  logicop=AND  UseBitMask=on  BitMask=0xF  BitMaskRealWorld=Stored Integer
  Bitwise AND2 : simulink/Logic and Bit Operations/Bitwise Operator  logicop=AND  UseBitMask=on  BitMask=0xFF0  BitMaskRealWorld=Stored Integer
  Bitwise AND3 : simulink/Logic and Bit Operations/Bitwise Operator  logicop=AND  UseBitMask=on  BitMask=0xFF  BitMaskRealWorld=Stored Integer
  Bitwise AND4 : simulink/Logic and Bit Operations/Bitwise Operator  logicop=AND  UseBitMask=on  BitMask=0xF00  BitMaskRealWorld=Stored Integer
  Bitwise AND5 : simulink/Logic and Bit Operations/Bitwise Operator  logicop=OR  UseBitMask=off  NumInputPorts=2  BitMask=0xFF  BitMaskRealWorld=Stored Integer
  Data Type Conversion1 : DataTypeConversion  OutDataTypeStr=uint8
  Data Type Conversion2 : DataTypeConversion  OutDataTypeStr=uint16
  Data Type Conversion3 : DataTypeConversion  OutDataTypeStr=uint8
  Data Type Conversion4 : DataTypeConversion  OutDataTypeStr=uint16
  Data Type Conversion5 : DataTypeConversion  OutDataTypeStr=uint8
  Gain : Gain  Gain=1/20
  Gain1 : Gain  Gain=1/40
  Mux2 : Mux  Inputs=3
  Shift Arithmetic1 : ArithShift  BitShiftNumber=8  BitShiftDirection=Right
  Shift Arithmetic2 : ArithShift  BitShiftNumber=4  BitShiftDirection=Left
  Shift Arithmetic39 : ArithShift  BitShiftNumber=4  BitShiftDirection=Right
  convert_out1 : FVT_lib/hal/convert_out  gain=0.001  offset=0
  convert_out4 : FVT_lib/hal/convert_out  gain=0.001  offset=0
  PedalZP_raw8 : Outport
  wires:
  Data Type Conversion1/1 -> Mux2/2
  Bitwise AND5/1 -> Data Type Conversion1/1
  Shift Arithmetic1/1 -> Bitwise AND5/2
  Shift Arithmetic2/1 -> Bitwise AND5/1
  Gain1/1 -> convert_out1/1
  Gain/1 -> convert_out4/1
  EAPS1_pct/1 -> Gain/1
  convert_out4/1 -> Data Type Conversion2/1
  convert_out1/1 -> Data Type Conversion4/1
  EAPS2_pct/1 -> Gain1/1
  Bitwise AND3/1 -> Data Type Conversion3/1
  Bitwise AND4/1 -> Shift Arithmetic1/1
  Data Type Conversion4/1 -> Bitwise AND3/1, Bitwise AND4/1
  Data Type Conversion3/1 -> Mux2/3
  Data Type Conversion5/1 -> Mux2/1
  Data Type Conversion2/1 -> Bitwise AND2/1, Bitwise AND1/1
  Bitwise AND2/1 -> Shift Arithmetic39/1
  Shift Arithmetic39/1 -> Data Type Conversion5/1
  Mux2/1 -> PedalZP_raw8/1
  Bitwise AND1/1 -> Shift Arithmetic2/1

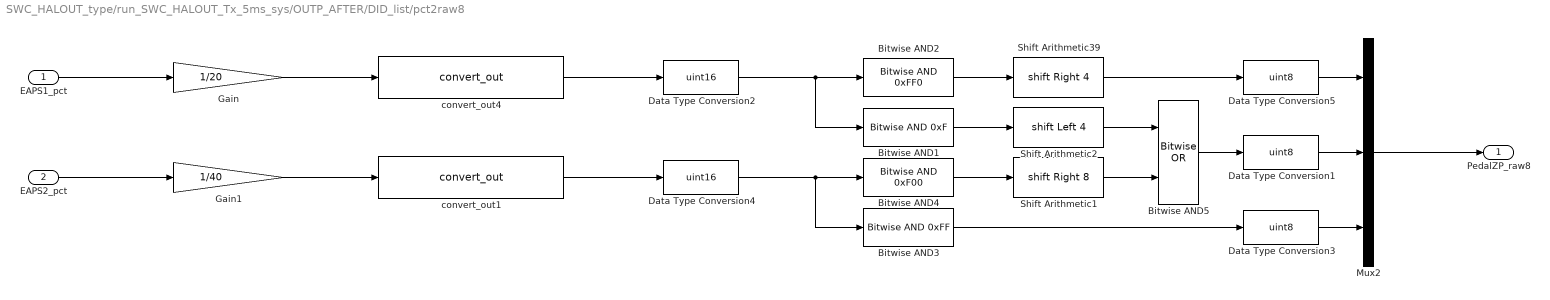
== system SWC_HALOUT_type/run_SWC_HALOUT_Tx_5ms_sys/OUTP_AFTER/DID_list/pct2raw8 ==
  EAPS1_pct : Inport
  EAPS2_pct : Inport  Port=2
  Bitwise AND1 : simulink/Logic and Bit Operations/Bitwise Operator  logicop=AND  UseBitMask=on  BitMask=0xF  BitMaskRealWorld=Stored Integer
  Bitwise AND2 : simulink/Logic and Bit Operations/Bitwise Operator  logicop=AND  UseBitMask=on  BitMask=0xFF0  BitMaskRealWorld=Stored Integer
  Bitwise AND3 : simulink/Logic and Bit Operations/Bitwise Operator  logicop=AND  UseBitMask=on  BitMask=0xFF  BitMaskRealWorld=Stored Integer
  Bitwise AND4 : simulink/Logic and Bit Operations/Bitwise Operator  logicop=AND  UseBitMask=on  BitMask=0xF00  BitMaskRealWorld=Stored Integer
  Bitwise AND5 : simulink/Logic and Bit Operations/Bitwise Operator  logicop=OR  UseBitMask=off  NumInputPorts=2  BitMask=0xFF  BitMaskRealWorld=Stored Integer
  Data Type Conversion1 : DataTypeConversion  OutDataTypeStr=uint8
  Data Type Conversion2 : DataTypeConversion  OutDataTypeStr=uint16
  Data Type Conversion3 : DataTypeConversion  OutDataTypeStr=uint8
  Data Type Conversion4 : DataTypeConversion  OutDataTypeStr=uint16
  Data Type Conversion5 : DataTypeConversion  OutDataTypeStr=uint8
  Gain : Gain  Gain=1/20
  Gain1 : Gain  Gain=1/40
  Mux2 : Mux  Inputs=3
  Shift Arithmetic1 : ArithShift  BitShiftNumber=8  BitShiftDirection=Right
  Shift Arithmetic2 : ArithShift  BitShiftNumber=4  BitShiftDirection=Left
  Shift Arithmetic39 : ArithShift  BitShiftNumber=4  BitShiftDirection=Right
  convert_out1 : FVT_lib/hal/convert_out  gain=0.001  offset=0
  convert_out4 : FVT_lib/hal/convert_out  gain=0.001  offset=0
  PedalZP_raw8 : Outport
  wires:
  Bitwise AND1/1 -> Shift Arithmetic2/1
  Mux2/1 -> PedalZP_raw8/1
  Shift Arithmetic39/1 -> Data Type Conversion5/1
  Bitwise AND2/1 -> Shift Arithmetic39/1
  Data Type Conversion2/1 -> Bitwise AND1/1, Bitwise AND2/1
  Data Type Conversion5/1 -> Mux2/1
  Data Type Conversion3/1 -> Mux2/3
  Data Type Conversion4/1 -> Bitwise AND4/1, Bitwise AND3/1
  Bitwise AND4/1 -> Shift Arithmetic1/1
  Bitwise AND3/1 -> Data Type Conversion3/1
  EAPS2_pct/1 -> Gain1/1
  convert_out1/1 -> Data Type Conversion4/1
  convert_out4/1 -> Data Type Conversion2/1
  EAPS1_pct/1 -> Gain/1
  Gain/1 -> convert_out4/1
  Gain1/1 -> convert_out1/1
  Shift Arithmetic2/1 -> Bitwise AND5/1
  Shift Arithmetic1/1 -> Bitwise AND5/2
  Bitwise AND5/1 -> Data Type Conversion1/1
  Data Type Conversion1/1 -> Mux2/2

== system SWC_HALOUT_type/run_SWC_HALOUT_Tx_5ms_sys/OUTP_AFTER/DID_list/uint32Touint8Array ==
  In1 : Inport
  Bitwise AND1 : simulink/Logic and Bit Operations/Bitwise Operator  logicop=AND  UseBitMask=on  BitMask=bin2dec('00000000000000000000000011111111')  BitMaskRealWorld=Stored Integer
  Bitwise AND2 : simulink/Logic and Bit Operations/Bitwise Operator  logicop=AND  UseBitMask=on  BitMask=bin2dec('00000000000000001111111100000000')  BitMaskRealWorld=Stored Integer
  Bitwise AND3 : simulink/Logic and Bit Operations/Bitwise Operator  logicop=AND  UseBitMask=on  BitMask=bin2dec('00000000111111110000000000000000')  BitMaskRealWorld=Stored Integer
  Bitwise AND4 : simulink/Logic and Bit Operations/Bitwise Operator  logicop=AND  UseBitMask=on  BitMask=bin2dec('11111111000000000000000000000000')  BitMaskRealWorld=Stored Integer
  Data Type Conversion{1,3..5} (4 alike) : DataTypeConversion  OutDataTypeStr=uint8
  Data Type Conversion2 : DataTypeConversion  OutDataTypeStr=uint32
  Mux2 : Mux
  Shift Arithmetic39 : ArithShift  BitShiftNumber=8  BitShiftDirection=Right
  Shift Arithmetic40 : ArithShift  BitShiftNumber=16  BitShiftDirection=Right
  Shift Arithmetic41 : ArithShift  BitShiftNumber=24  BitShiftDirection=Right
  Out1 : Outport
  wires:
  Bitwise AND4/1 -> Shift Arithmetic41/1
  Bitwise AND1/1 -> Data Type Conversion1/1
  Shift Arithmetic40/1 -> Data Type Conversion4/1
  Shift Arithmetic41/1 -> Data Type Conversion3/1
  Mux2/1 -> Out1/1
  In1/1 -> Data Type Conversion2/1
  Bitwise AND3/1 -> Shift Arithmetic40/1
  Shift Arithmetic39/1 -> Data Type Conversion5/1
  Data Type Conversion3/1 -> Mux2/1
  Bitwise AND2/1 -> Shift Arithmetic39/1
  Data Type Conversion2/1 -> Bitwise AND4/1, Bitwise AND3/1, Bitwise AND1/1, Bitwise AND2/1
  Data Type Conversion5/1 -> Mux2/3
  Data Type Conversion4/1 -> Mux2/2
  Data Type Conversion1/1 -> Mux2/4

== system SWC_HALOUT_type/run_SWC_HALOUT_Tx_5ms_sys/OUTP_AFTER/DID_list/uint32Touint8Array1 ==
  In1 : Inport
  Bitwise AND1 : simulink/Logic and Bit Operations/Bitwise Operator  logicop=AND  UseBitMask=on  BitMask=bin2dec('00000000000000000000000011111111')  BitMaskRealWorld=Stored Integer
  Bitwise AND2 : simulink/Logic and Bit Operations/Bitwise Operator  logicop=AND  UseBitMask=on  BitMask=bin2dec('00000000000000001111111100000000')  BitMaskRealWorld=Stored Integer
  Bitwise AND3 : simulink/Logic and Bit Operations/Bitwise Operator  logicop=AND  UseBitMask=on  BitMask=bin2dec('00000000111111110000000000000000')  BitMaskRealWorld=Stored Integer
  Bitwise AND4 : simulink/Logic and Bit Operations/Bitwise Operator  logicop=AND  UseBitMask=on  BitMask=bin2dec('11111111000000000000000000000000')  BitMaskRealWorld=Stored Integer
  Data Type Conversion{1,3..5} (4 alike) : DataTypeConversion  OutDataTypeStr=uint8
  Data Type Conversion2 : DataTypeConversion  OutDataTypeStr=uint32
  Mux2 : Mux
  Shift Arithmetic39 : ArithShift  BitShiftNumber=8  BitShiftDirection=Right
  Shift Arithmetic40 : ArithShift  BitShiftNumber=16  BitShiftDirection=Right
  Shift Arithmetic41 : ArithShift  BitShiftNumber=24  BitShiftDirection=Right
  Out1 : Outport
  wires:
  Data Type Conversion1/1 -> Mux2/4
  Data Type Conversion4/1 -> Mux2/2
  Data Type Conversion5/1 -> Mux2/3
  Data Type Conversion2/1 -> Bitwise AND2/1, Bitwise AND1/1, Bitwise AND3/1, Bitwise AND4/1
  Bitwise AND2/1 -> Shift Arithmetic39/1
  Data Type Conversion3/1 -> Mux2/1
  Shift Arithmetic39/1 -> Data Type Conversion5/1
  Bitwise AND3/1 -> Shift Arithmetic40/1
  In1/1 -> Data Type Conversion2/1
  Mux2/1 -> Out1/1
  Shift Arithmetic41/1 -> Data Type Conversion3/1
  Shift Arithmetic40/1 -> Data Type Conversion4/1
  Bitwise AND1/1 -> Data Type Conversion1/1
  Bitwise AND4/1 -> Shift Arithmetic41/1

== system SWC_HALOUT_type/run_SWC_HALOUT_Tx_5ms_sys/OUTP_AFTER/DID_list/uint32Touint8Array2 ==
  In1 : Inport
  Bitwise AND1 : simulink/Logic and Bit Operations/Bitwise Operator  logicop=AND  UseBitMask=on  BitMask=bin2dec('00000000000000000000000011111111')  BitMaskRealWorld=Stored Integer
  Bitwise AND2 : simulink/Logic and Bit Operations/Bitwise Operator  logicop=AND  UseBitMask=on  BitMask=bin2dec('00000000000000001111111100000000')  BitMaskRealWorld=Stored Integer
  Bitwise AND3 : simulink/Logic and Bit Operations/Bitwise Operator  logicop=AND  UseBitMask=on  BitMask=bin2dec('00000000111111110000000000000000')  BitMaskRealWorld=Stored Integer
  Bitwise AND4 : simulink/Logic and Bit Operations/Bitwise Operator  logicop=AND  UseBitMask=on  BitMask=bin2dec('11111111000000000000000000000000')  BitMaskRealWorld=Stored Integer
  Data Type Conversion{1,3..5} (4 alike) : DataTypeConversion  OutDataTypeStr=uint8
  Data Type Conversion2 : DataTypeConversion  OutDataTypeStr=uint32
  Mux2 : Mux
  Shift Arithmetic39 : ArithShift  BitShiftNumber=8  BitShiftDirection=Right
  Shift Arithmetic40 : ArithShift  BitShiftNumber=16  BitShiftDirection=Right
  Shift Arithmetic41 : ArithShift  BitShiftNumber=24  BitShiftDirection=Right
  Out1 : Outport
  wires:
  Bitwise AND4/1 -> Shift Arithmetic41/1
  Bitwise AND1/1 -> Data Type Conversion1/1
  Shift Arithmetic40/1 -> Data Type Conversion4/1
  Shift Arithmetic41/1 -> Data Type Conversion3/1
  Mux2/1 -> Out1/1
  In1/1 -> Data Type Conversion2/1
  Bitwise AND3/1 -> Shift Arithmetic40/1
  Shift Arithmetic39/1 -> Data Type Conversion5/1
  Data Type Conversion3/1 -> Mux2/1
  Bitwise AND2/1 -> Shift Arithmetic39/1
  Data Type Conversion2/1 -> Bitwise AND4/1, Bitwise AND3/1, Bitwise AND1/1, Bitwise AND2/1
  Data Type Conversion5/1 -> Mux2/3
  Data Type Conversion4/1 -> Mux2/2
  Data Type Conversion1/1 -> Mux2/4

== system SWC_HALOUT_type/run_SWC_HALOUT_Tx_5ms_sys/OUTP_AFTER/DID_list/uint32Touint8Array3 ==
  In1 : Inport
  Bitwise AND1 : simulink/Logic and Bit Operations/Bitwise Operator  logicop=AND  UseBitMask=on  BitMask=bin2dec('00000000000000000000000011111111')  BitMaskRealWorld=Stored Integer
  Bitwise AND2 : simulink/Logic and Bit Operations/Bitwise Operator  logicop=AND  UseBitMask=on  BitMask=bin2dec('00000000000000001111111100000000')  BitMaskRealWorld=Stored Integer
  Bitwise AND3 : simulink/Logic and Bit Operations/Bitwise Operator  logicop=AND  UseBitMask=on  BitMask=bin2dec('00000000111111110000000000000000')  BitMaskRealWorld=Stored Integer
  Bitwise AND4 : simulink/Logic and Bit Operations/Bitwise Operator  logicop=AND  UseBitMask=on  BitMask=bin2dec('11111111000000000000000000000000')  BitMaskRealWorld=Stored Integer
  Data Type Conversion{1,3..5} (4 alike) : DataTypeConversion  OutDataTypeStr=uint8
  Data Type Conversion2 : DataTypeConversion  OutDataTypeStr=uint32
  Mux2 : Mux
  Shift Arithmetic39 : ArithShift  BitShiftNumber=8  BitShiftDirection=Right
  Shift Arithmetic40 : ArithShift  BitShiftNumber=16  BitShiftDirection=Right
  Shift Arithmetic41 : ArithShift  BitShiftNumber=24  BitShiftDirection=Right
  Out1 : Outport
  wires:
  Data Type Conversion1/1 -> Mux2/4
  Data Type Conversion4/1 -> Mux2/2
  Data Type Conversion5/1 -> Mux2/3
  Data Type Conversion2/1 -> Bitwise AND2/1, Bitwise AND1/1, Bitwise AND3/1, Bitwise AND4/1
  Bitwise AND2/1 -> Shift Arithmetic39/1
  Data Type Conversion3/1 -> Mux2/1
  Shift Arithmetic39/1 -> Data Type Conversion5/1
  Bitwise AND3/1 -> Shift Arithmetic40/1
  In1/1 -> Data Type Conversion2/1
  Mux2/1 -> Out1/1
  Shift Arithmetic41/1 -> Data Type Conversion3/1
  Shift Arithmetic40/1 -> Data Type Conversion4/1
  Bitwise AND1/1 -> Data Type Conversion1/1
  Bitwise AND4/1 -> Shift Arithmetic41/1
